simulink model "Ampl_modl"  (R2020a)
settings: Solver=VariableStepAuto  StartTime=0.0  StopTime=10  MaxStep=0.001  RelTol=1e-3
settings Model: NumberOfSteps=5  Creator=Atharv Sharma  LastModifiedBy=Atharv Sharma

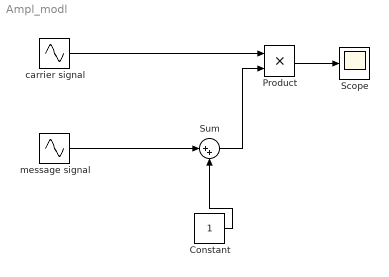
== system Ampl_modl ==
  Constant : Constant
  Product : Product
  Scope : Scope
  Sum : Sum  Inputs=|++
  carrier signal : Sin  Frequency=1000  SampleTime=0
  message signal : Sin  Amplitude=.5  Frequency=10  SampleTime=0
  wires:
  Constant/1 -> Sum/2
  message signal/1 -> Sum/1
  Sum/1 -> Product/2
  carrier signal/1 -> Product/1
  Product/1 -> Scope/1
